simulink library "halin"  (R2021b)
settings: Solver=VariableStepAuto  StartTime=0.0  StopTime=10.0  RelTol=1e-3
undefined symbols (not defined in the file): TRUE
libraries: FVT_lib x177, hcu_lib x55
(part 14 of 17)

== system halin/HAL_IN/CAN2/IVI3/IVICLBlowerYSta ==
  IVI_CLBlower_Y_Sta : Inport
  UnitConverter : DataTypeConversion  OutDataTypeStr=uint8
  VHAL_IVICLBlowerYSta_pct : Outport
  wires:
  UnitConverter/1 -> VHAL_IVICLBlowerYSta_pct/1
  IVI_CLBlower_Y_Sta/1 -> UnitConverter/1

== system halin/HAL_IN/CAN2/IVI3/IVICLBlowerZSta ==
  IVI_CLBlower_Z_Sta : Inport
  UnitConverter : DataTypeConversion  OutDataTypeStr=uint8
  VHAL_IVICLBlowerZSta_pct : Outport
  wires:
  UnitConverter/1 -> VHAL_IVICLBlowerZSta_pct/1
  IVI_CLBlower_Z_Sta/1 -> UnitConverter/1

== system halin/HAL_IN/CAN2/IVI3/IVICRBlowerYSta ==
  IVI_CRBlower_Y_Sta : Inport
  UnitConverter : DataTypeConversion  OutDataTypeStr=uint8
  VHAL_IVICRBlowerYSta_pct : Outport
  wires:
  UnitConverter/1 -> VHAL_IVICRBlowerYSta_pct/1
  IVI_CRBlower_Y_Sta/1 -> UnitConverter/1

== system halin/HAL_IN/CAN2/IVI3/IVICRBlowerZSta ==
  IVI_CRBlower_Z_Sta : Inport
  UnitConverter : DataTypeConversion  OutDataTypeStr=uint8
  VHAL_IVICRBlowerZSta_pct : Outport
  wires:
  UnitConverter/1 -> VHAL_IVICRBlowerZSta_pct/1
  IVI_CRBlower_Z_Sta/1 -> UnitConverter/1

== system halin/HAL_IN/CAN2/IVI3/IVIDrBlowerModeSta ==
  IVI_DrBlower_Mode_Sta : Inport
  UnitConverter : DataTypeConversion  OutDataTypeStr=uint8
  VHAL_IVIDrBlowerModeSta_enum : Outport
  wires:
  UnitConverter/1 -> VHAL_IVIDrBlowerModeSta_enum/1
  IVI_DrBlower_Mode_Sta/1 -> UnitConverter/1

== system halin/HAL_IN/CAN2/IVI3/IVIDrBlowerYSta ==
  IVI_DrBlower_Y_Sta : Inport
  UnitConverter : DataTypeConversion  OutDataTypeStr=uint8
  VHAL_IVIDrBlowerYSta_pct : Outport
  wires:
  UnitConverter/1 -> VHAL_IVIDrBlowerYSta_pct/1
  IVI_DrBlower_Y_Sta/1 -> UnitConverter/1

== system halin/HAL_IN/CAN2/IVI3/IVIDrBlowerZSta ==
  IVI_DrBlower_Z_Sta : Inport
  UnitConverter : DataTypeConversion  OutDataTypeStr=uint8
  VHAL_IVIDrBlowerZSta_pct : Outport
  wires:
  UnitConverter/1 -> VHAL_IVIDrBlowerZSta_pct/1
  IVI_DrBlower_Z_Sta/1 -> UnitConverter/1

== system halin/HAL_IN/CAN2/IVI3/IVILSEATventCmd ==
  IVI_LSEATvent_Cmd : Inport
  UnitConverter : DataTypeConversion  OutDataTypeStr=uint8
  VHAL_IVILSEATventCmd_enum : Outport
  wires:
  UnitConverter/1 -> VHAL_IVILSEATventCmd_enum/1
  IVI_LSEATvent_Cmd/1 -> UnitConverter/1

== system halin/HAL_IN/CAN2/IVI3/IVIMLFMostCmd ==
  IVI_MLFMost_Cmd : Inport
  UnitConverter : DataTypeConversion  OutDataTypeStr=uint8
  VHAL_IVIMLFMostCmd_flg : Outport
  wires:
  UnitConverter/1 -> VHAL_IVIMLFMostCmd_flg/1
  IVI_MLFMost_Cmd/1 -> UnitConverter/1

== system halin/HAL_IN/CAN2/IVI3/IVIMLFootLiftCmd ==
  IVI_MLFootLift_Cmd : Inport
  UnitConverter : DataTypeConversion  OutDataTypeStr=uint8
  VHAL_IVIMLFootLiftCmd_enum : Outport
  wires:
  UnitConverter/1 -> VHAL_IVIMLFootLiftCmd_enum/1
  IVI_MLFootLift_Cmd/1 -> UnitConverter/1

== system halin/HAL_IN/CAN2/IVI3/IVIMLNapModeCmd ==
  IVI_MLNapMode_Cmd : Inport
  UnitConverter : DataTypeConversion  OutDataTypeStr=uint8
  VHAL_IVIMLNapModeCmd_flg : Outport
  wires:
  UnitConverter/1 -> VHAL_IVIMLNapModeCmd_flg/1
  IVI_MLNapMode_Cmd/1 -> UnitConverter/1

== system halin/HAL_IN/CAN2/IVI3/IVIMLReclinerCmd ==
  IVI_MLRecliner_Cmd : Inport
  UnitConverter : DataTypeConversion  OutDataTypeStr=uint8
  VHAL_IVIMLReclinerCmd_enum : Outport
  wires:
  UnitConverter/1 -> VHAL_IVIMLReclinerCmd_enum/1
  IVI_MLRecliner_Cmd/1 -> UnitConverter/1

== system halin/HAL_IN/CAN2/IVI3/IVIMLRestoreCmd ==
  IVI_MLRestore_Cmd : Inport
  UnitConverter : DataTypeConversion  OutDataTypeStr=uint8
  VHAL_IVIMLRestoreCmd_flg : Outport
  wires:
  UnitConverter/1 -> VHAL_IVIMLRestoreCmd_flg/1
  IVI_MLRestore_Cmd/1 -> UnitConverter/1

== system halin/HAL_IN/CAN2/IVI3/IVIMLSEATventCmd ==
  IVI_MLSEATvent_Cmd : Inport
  UnitConverter : DataTypeConversion  OutDataTypeStr=uint8
  VHAL_IVIMLSEATventCmd_enum : Outport
  wires:
  UnitConverter/1 -> VHAL_IVIMLSEATventCmd_enum/1
  IVI_MLSEATvent_Cmd/1 -> UnitConverter/1

== system halin/HAL_IN/CAN2/IVI3/IVIMLSeatLiftCmd ==
  IVI_MLSeatLift_Cmd : Inport
  UnitConverter : DataTypeConversion  OutDataTypeStr=uint8
  VHAL_IVIMLSeatLiftCmd_enum : Outport
  wires:
  UnitConverter/1 -> VHAL_IVIMLSeatLiftCmd_enum/1
  IVI_MLSeatLift_Cmd/1 -> UnitConverter/1

== system halin/HAL_IN/CAN2/IVI3/IVIMLSldRestoreCmd ==
  IVI_MLSldRestore_Cmd : Inport
  UnitConverter : DataTypeConversion  OutDataTypeStr=uint8
  VHAL_IVIMLSldRestoreCmd_flg : Outport
  wires:
  UnitConverter/1 -> VHAL_IVIMLSldRestoreCmd_flg/1
  IVI_MLSldRestore_Cmd/1 -> UnitConverter/1

== system halin/HAL_IN/CAN2/IVI3/IVIMLSliderCmd ==
  IVI_MLSlider_Cmd : Inport
  UnitConverter : DataTypeConversion  OutDataTypeStr=uint8
  VHAL_IVIMLSliderCmd_enum : Outport
  wires:
  UnitConverter/1 -> VHAL_IVIMLSliderCmd_enum/1
  IVI_MLSlider_Cmd/1 -> UnitConverter/1

== system halin/HAL_IN/CAN2/IVI3/IVIMLZeroGravityCmd ==
  IVI_MLZeroGravity_Cmd : Inport
  UnitConverter : DataTypeConversion  OutDataTypeStr=uint8
  VHAL_IVIMLZeroGravityCmd_flg : Outport
  wires:
  UnitConverter/1 -> VHAL_IVIMLZeroGravityCmd_flg/1
  IVI_MLZeroGravity_Cmd/1 -> UnitConverter/1

== system halin/HAL_IN/CAN2/IVI3/IVIMRFMostCmd ==
  IVI_MRFMost_Cmd : Inport
  UnitConverter : DataTypeConversion  OutDataTypeStr=uint8
  VHAL_IVIMRFMostCmd_flg : Outport
  wires:
  UnitConverter/1 -> VHAL_IVIMRFMostCmd_flg/1
  IVI_MRFMost_Cmd/1 -> UnitConverter/1

== system halin/HAL_IN/CAN2/IVI3/IVIMRFootLiftCmd ==
  IVI_MRFootLift_Cmd : Inport
  UnitConverter : DataTypeConversion  OutDataTypeStr=uint8
  VHAL_IVIMRFootLiftCmd_enum : Outport
  wires:
  UnitConverter/1 -> VHAL_IVIMRFootLiftCmd_enum/1
  IVI_MRFootLift_Cmd/1 -> UnitConverter/1

== system halin/HAL_IN/CAN2/IVI3/IVIMRNapModeCmd ==
  IVI_MRNapMode_Cmd : Inport
  UnitConverter : DataTypeConversion  OutDataTypeStr=uint8
  VHAL_IVIMRNapModeCmd_flg : Outport
  wires:
  UnitConverter/1 -> VHAL_IVIMRNapModeCmd_flg/1
  IVI_MRNapMode_Cmd/1 -> UnitConverter/1

== system halin/HAL_IN/CAN2/IVI3/IVIMRReclinerCmd ==
  IVI_MRRecliner_Cmd : Inport
  UnitConverter : DataTypeConversion  OutDataTypeStr=uint8
  VHAL_IVIMRReclinerCmd_enum : Outport
  wires:
  UnitConverter/1 -> VHAL_IVIMRReclinerCmd_enum/1
  IVI_MRRecliner_Cmd/1 -> UnitConverter/1

== system halin/HAL_IN/CAN2/IVI3/IVIMRRestoreCmd ==
  IVI_MRRestore_Cmd : Inport
  UnitConverter : DataTypeConversion  OutDataTypeStr=uint8
  VHAL_IVIMRRestoreCmd_flg : Outport
  wires:
  UnitConverter/1 -> VHAL_IVIMRRestoreCmd_flg/1
  IVI_MRRestore_Cmd/1 -> UnitConverter/1

== system halin/HAL_IN/CAN2/IVI3/IVIMRSEATventCmd ==
  IVI_MRSEATvent_Cmd : Inport
  UnitConverter : DataTypeConversion  OutDataTypeStr=uint8
  VHAL_IVIMRSEATventCmd_enum : Outport
  wires:
  UnitConverter/1 -> VHAL_IVIMRSEATventCmd_enum/1
  IVI_MRSEATvent_Cmd/1 -> UnitConverter/1

== system halin/HAL_IN/CAN2/IVI3/IVIMRSeatLiftCmd ==
  IVI_MRSeatLift_Cmd : Inport
  UnitConverter : DataTypeConversion  OutDataTypeStr=uint8
  VHAL_IVIMRSeatLiftCmd_enum : Outport
  wires:
  UnitConverter/1 -> VHAL_IVIMRSeatLiftCmd_enum/1
  IVI_MRSeatLift_Cmd/1 -> UnitConverter/1

== system halin/HAL_IN/CAN2/IVI3/IVIMRSldRestoreCmd ==
  IVI_MRSldRestore_Cmd : Inport
  UnitConverter : DataTypeConversion  OutDataTypeStr=uint8
  VHAL_IVIMRSldRestoreCmd_flg : Outport
  wires:
  UnitConverter/1 -> VHAL_IVIMRSldRestoreCmd_flg/1
  IVI_MRSldRestore_Cmd/1 -> UnitConverter/1

== system halin/HAL_IN/CAN2/IVI3/IVIMRSliderCmd ==
  IVI_MRSlider_Cmd : Inport
  UnitConverter : DataTypeConversion  OutDataTypeStr=uint8
  VHAL_IVIMRSliderCmd_enum : Outport
  wires:
  UnitConverter/1 -> VHAL_IVIMRSliderCmd_enum/1
  IVI_MRSlider_Cmd/1 -> UnitConverter/1

== system halin/HAL_IN/CAN2/IVI3/IVIMRZeroGravityCmd ==
  IVI_MRZeroGravity_Cmd : Inport
  UnitConverter : DataTypeConversion  OutDataTypeStr=uint8
  VHAL_IVIMRZeroGravityCmd_flg : Outport
  wires:
  UnitConverter/1 -> VHAL_IVIMRZeroGravityCmd_flg/1
  IVI_MRZeroGravity_Cmd/1 -> UnitConverter/1

== system halin/HAL_IN/CAN2/IVI3/IVIPsBlowerModeSta ==
  IVI_PsBlower_Mode_Sta : Inport
  UnitConverter : DataTypeConversion  OutDataTypeStr=uint8
  VHAL_IVIPsBlowerModeSta_enum : Outport
  wires:
  UnitConverter/1 -> VHAL_IVIPsBlowerModeSta_enum/1
  IVI_PsBlower_Mode_Sta/1 -> UnitConverter/1

== system halin/HAL_IN/CAN2/IVI3/IVIPsBlowerYSta ==
  IVI_PsBlower_Y_Sta : Inport
  UnitConverter : DataTypeConversion  OutDataTypeStr=uint8
  VHAL_IVIPsBlowerYSta_pct : Outport
  wires:
  UnitConverter/1 -> VHAL_IVIPsBlowerYSta_pct/1
  IVI_PsBlower_Y_Sta/1 -> UnitConverter/1

== system halin/HAL_IN/CAN2/IVI3/IVIPsBlowerZSta ==
  IVI_PsBlower_Z_Sta : Inport
  UnitConverter : DataTypeConversion  OutDataTypeStr=uint8
  VHAL_IVIPsBlowerZSta_pct : Outport
  wires:
  UnitConverter/1 -> VHAL_IVIPsBlowerZSta_pct/1
  IVI_PsBlower_Z_Sta/1 -> UnitConverter/1

== system halin/HAL_IN/CAN2/IVI3/IVIRSEATventCmd ==
  IVI_RSEATvent_Cmd : Inport
  UnitConverter : DataTypeConversion  OutDataTypeStr=uint8
  VHAL_IVIRSEATventCmd_enum : Outport
  wires:
  UnitConverter/1 -> VHAL_IVIRSEATventCmd_enum/1
  IVI_RSEATvent_Cmd/1 -> UnitConverter/1

== system halin/HAL_IN/CAN2/METER1/METERKPHCalcu ==
  METER_KPH_Calcu : Inport
  UnitConverter : DataTypeConversion  OutDataTypeStr=uint8
  VHAL_METERKPHCalcu_kph : Outport
  wires:
  UnitConverter/1 -> VHAL_METERKPHCalcu_kph/1
  METER_KPH_Calcu/1 -> UnitConverter/1

== system halin/HAL_IN/CAN2/METER1/ODOMETER ==
  ODOMETER : Inport
  UnitConverter : DataTypeConversion  OutDataTypeStr=uint32
  convert_in : FVT_lib/hal/convert_in  gain=0.1  offset=0
  VHAL_ODOMETER_km : Outport
  wires:
  convert_in/1 -> VHAL_ODOMETER_km/1
  UnitConverter/1 -> convert_in/1
  ODOMETER/1 -> UnitConverter/1

== system halin/HAL_IN/CAN3/BMS1/BMSChckSum1 ==
  BMSChckSum_1 : Inport
  UnitConverter : DataTypeConversion  OutDataTypeStr=uint8
  VHAL_BMSChckSum1_enum : Outport
  wires:
  UnitConverter/1 -> VHAL_BMSChckSum1_enum/1
  BMSChckSum_1/1 -> UnitConverter/1

== system halin/HAL_IN/CAN3/BMS1/BMSRolCnct1 ==
  BMSRolCnct_1 : Inport
  UnitConverter : DataTypeConversion  OutDataTypeStr=uint8
  VHAL_BMSRolCnct1_enum : Outport
  wires:
  UnitConverter/1 -> VHAL_BMSRolCnct1_enum/1
  BMSRolCnct_1/1 -> UnitConverter/1

== system halin/HAL_IN/CAN3/BMS1/HVBPwrAvailChrg ==
  HVBPwrAvailChrg : Inport
  UnitConverter : DataTypeConversion  OutDataTypeStr=uint16
  convert_in : FVT_lib/hal/convert_in  gain=0.2  offset=0
  VHAL_HVBPwrAvailChrg_kW : Outport
  wires:
  convert_in/1 -> VHAL_HVBPwrAvailChrg_kW/1
  UnitConverter/1 -> convert_in/1
  HVBPwrAvailChrg/1 -> UnitConverter/1

== system halin/HAL_IN/CAN3/BMS1/HVBPwrAvailChrg30 ==
  HVBPwrAvailChrg30 : Inport
  UnitConverter : DataTypeConversion  OutDataTypeStr=uint16
  convert_in : FVT_lib/hal/convert_in  gain=0.2  offset=0
  VHAL_HVBPwrAvailChrg30_kW : Outport
  wires:
  convert_in/1 -> VHAL_HVBPwrAvailChrg30_kW/1
  UnitConverter/1 -> convert_in/1
  HVBPwrAvailChrg30/1 -> UnitConverter/1

== system halin/HAL_IN/CAN3/BMS1/HVBPwrAvailChrg60 ==
  HVBPwrAvailChrg60 : Inport
  UnitConverter : DataTypeConversion  OutDataTypeStr=uint16
  convert_in : FVT_lib/hal/convert_in  gain=0.2  offset=0
  VHAL_HVBPwrAvailChrg60_kW : Outport
  wires:
  convert_in/1 -> VHAL_HVBPwrAvailChrg60_kW/1
  UnitConverter/1 -> convert_in/1
  HVBPwrAvailChrg60/1 -> UnitConverter/1

== system halin/HAL_IN/CAN3/BMS1/HVBPwrAvailDchrg ==
  HVBPwrAvailDchrg : Inport
  UnitConverter : DataTypeConversion  OutDataTypeStr=uint16
  convert_in : FVT_lib/hal/convert_in  gain=0.2  offset=0
  VHAL_HVBPwrAvailDchrg_kW : Outport
  wires:
  convert_in/1 -> VHAL_HVBPwrAvailDchrg_kW/1
  UnitConverter/1 -> convert_in/1
  HVBPwrAvailDchrg/1 -> UnitConverter/1

== system halin/HAL_IN/CAN3/BMS1/HVBPwrAvailDchrg30 ==
  HVBPwrAvailDchrg30 : Inport
  UnitConverter : DataTypeConversion  OutDataTypeStr=uint16
  convert_in : FVT_lib/hal/convert_in  gain=0.2  offset=0
  VHAL_HVBPwrAvailDchrg30_kW : Outport
  wires:
  convert_in/1 -> VHAL_HVBPwrAvailDchrg30_kW/1
  UnitConverter/1 -> convert_in/1
  HVBPwrAvailDchrg30/1 -> UnitConverter/1

== system halin/HAL_IN/CAN3/BMS1/HVBPwrAvailDchrg60 ==
  HVBPwrAvailDchrg60 : Inport
  UnitConverter : DataTypeConversion  OutDataTypeStr=uint16
  convert_in : FVT_lib/hal/convert_in  gain=0.2  offset=0
  VHAL_HVBPwrAvailDchrg60_kW : Outport
  wires:
  convert_in/1 -> VHAL_HVBPwrAvailDchrg60_kW/1
  UnitConverter/1 -> convert_in/1
  HVBPwrAvailDchrg60/1 -> UnitConverter/1

== system halin/HAL_IN/CAN3/BMS1/HVBattCurr ==
  HVBattCurr : Inport
  UnitConverter : DataTypeConversion  OutDataTypeStr=uint16
  convert_in : FVT_lib/hal/convert_in  gain=0.1  offset=-1000
  VHAL_HVBattCurr_A : Outport
  wires:
  convert_in/1 -> VHAL_HVBattCurr_A/1
  UnitConverter/1 -> convert_in/1
  HVBattCurr/1 -> UnitConverter/1

== system halin/HAL_IN/CAN3/BMS1/HVBattVolt ==
  HVBattVolt : Inport
  UnitConverter : DataTypeConversion  OutDataTypeStr=uint16
  convert_in : FVT_lib/hal/convert_in  gain=0.1  offset=0
  VHAL_HVBattVolt_V : Outport
  wires:
  convert_in/1 -> VHAL_HVBattVolt_V/1
  UnitConverter/1 -> convert_in/1
  HVBattVolt/1 -> UnitConverter/1

== system halin/HAL_IN/CAN3/BMS3/ACChrgCurrDis ==
  ACChrgCurrDis : Inport
  UnitConverter : DataTypeConversion  OutDataTypeStr=uint16
  convert_in : FVT_lib/hal/convert_in  gain=0.1  offset=-1000
  VHAL_ACChrgCurrDis_A : Outport
  wires:
  convert_in/1 -> VHAL_ACChrgCurrDis_A/1
  UnitConverter/1 -> convert_in/1
  ACChrgCurrDis/1 -> UnitConverter/1

== system halin/HAL_IN/CAN3/BMS3/FireDetErr ==
  FireDetErr : Inport
  UnitConverter : DataTypeConversion  OutDataTypeStr=uint8
  VHAL_FireDetErr_flg : Outport
  wires:
  UnitConverter/1 -> VHAL_FireDetErr_flg/1
  FireDetErr/1 -> UnitConverter/1

== system halin/HAL_IN/CAN3/BMS3/HVBChrgPwr ==
  HVBChrgPwr : Inport
  UnitConverter : DataTypeConversion  OutDataTypeStr=uint16
  convert_in : FVT_lib/hal/convert_in  gain=0.1  offset=0
  VHAL_HVBChrgPwr_kWh : Outport
  wires:
  convert_in/1 -> VHAL_HVBChrgPwr_kWh/1
  UnitConverter/1 -> convert_in/1
  HVBChrgPwr/1 -> UnitConverter/1

== system halin/HAL_IN/CAN3/BMS3/HVBChrgPwrTotal ==
  HVBChrgPwrTotal : Inport
  UnitConverter : DataTypeConversion  OutDataTypeStr=uint32
  VHAL_HVBChrgPwrTotal_kWh : Outport
  wires:
  UnitConverter/1 -> VHAL_HVBChrgPwrTotal_kWh/1
  HVBChrgPwrTotal/1 -> UnitConverter/1

== system halin/HAL_IN/CAN3/BMS3/HVBDrvPwr ==
  HVBDrvPwr : Inport
  UnitConverter : DataTypeConversion  OutDataTypeStr=uint16
  convert_in : FVT_lib/hal/convert_in  gain=0.1  offset=0
  VHAL_HVBDrvPwr_kWh : Outport
  wires:
  convert_in/1 -> VHAL_HVBDrvPwr_kWh/1
  UnitConverter/1 -> convert_in/1
  HVBDrvPwr/1 -> UnitConverter/1

== system halin/HAL_IN/CAN3/BMS3/HVBDrvPwrTotal ==
  HVBDrvPwrTotal : Inport
  UnitConverter : DataTypeConversion  OutDataTypeStr=uint32
  VHAL_HVBDrvPwrTotal_kWh : Outport
  wires:
  UnitConverter/1 -> VHAL_HVBDrvPwrTotal_kWh/1
  HVBDrvPwrTotal/1 -> UnitConverter/1

== system halin/HAL_IN/CAN3/BMS3/HVBFullChrgPwr ==
  HVBFullChrgPwr : Inport
  UnitConverter : DataTypeConversion  OutDataTypeStr=uint16
  convert_in : FVT_lib/hal/convert_in  gain=0.1  offset=0
  VHAL_HVBFullChrgPwr_kWh : Outport
  wires:
  convert_in/1 -> VHAL_HVBFullChrgPwr_kWh/1
  UnitConverter/1 -> convert_in/1
  HVBFullChrgPwr/1 -> UnitConverter/1

== system halin/HAL_IN/CAN3/BMS3/HVBIsoImpedenceN ==
  HVBIsoImpedenceN : Inport
  UnitConverter : DataTypeConversion  OutDataTypeStr=uint16
  convert_in : FVT_lib/hal/convert_in  gain=0.01  offset=0
  VHAL_HVBIsoImpedenceN_Megaohm : Outport
  wires:
  convert_in/1 -> VHAL_HVBIsoImpedenceN_Megaohm/1
  UnitConverter/1 -> convert_in/1
  HVBIsoImpedenceN/1 -> UnitConverter/1

== system halin/HAL_IN/CAN3/BMS3/HVBIsoImpedenceP ==
  HVBIsoImpedenceP : Inport
  UnitConverter : DataTypeConversion  OutDataTypeStr=uint16
  convert_in : FVT_lib/hal/convert_in  gain=0.01  offset=0
  VHAL_HVBIsoImpedenceP_Megaohm : Outport
  wires:
  convert_in/1 -> VHAL_HVBIsoImpedenceP_Megaohm/1
  UnitConverter/1 -> convert_in/1
  HVBIsoImpedenceP/1 -> UnitConverter/1

== system halin/HAL_IN/CAN3/BMS3/HVBSOH ==
  HVBSOH : Inport
  UnitConverter : DataTypeConversion  OutDataTypeStr=uint8
  convert_in : FVT_lib/hal/convert_in  gain=0.4  offset=0
  VHAL_HVBSOH_pct : Outport
  wires:
  convert_in/1 -> VHAL_HVBSOH_pct/1
  UnitConverter/1 -> convert_in/1
  HVBSOH/1 -> UnitConverter/1

== system halin/HAL_IN/CAN3/BMS3/HVBattErr ==
  HVBattErr : Inport
  UnitConverter : DataTypeConversion  OutDataTypeStr=uint8
  VHAL_HVBattErr_flg : Outport
  wires:
  UnitConverter/1 -> VHAL_HVBattErr_flg/1
  HVBattErr/1 -> UnitConverter/1

== system halin/HAL_IN/CAN3/BMS3/HVBattPackVolt ==
  HVBattPackVolt : Inport
  UnitConverter : DataTypeConversion  OutDataTypeStr=uint16
  convert_in : FVT_lib/hal/convert_in  gain=0.1  offset=0
  VHAL_HVBattPackVolt_V : Outport
  wires:
  convert_in/1 -> VHAL_HVBattPackVolt_V/1
  UnitConverter/1 -> convert_in/1
  HVBattPackVolt/1 -> UnitConverter/1

== system halin/HAL_IN/CAN3/BMS3/HVBattSOC ==
  HVBattSOC : Inport
  UnitConverter : DataTypeConversion  OutDataTypeStr=uint8
  convert_in : FVT_lib/hal/convert_in  gain=0.4  offset=0
  VHAL_HVBattSOC_pct : Outport
  wires:
  convert_in/1 -> VHAL_HVBattSOC_pct/1
  UnitConverter/1 -> convert_in/1
  HVBattSOC/1 -> UnitConverter/1

== system halin/HAL_IN/CAN3/BMS3/HVBattSOCDis ==
  HVBattSOCDis : Inport
  UnitConverter : DataTypeConversion  OutDataTypeStr=uint8
  convert_in : FVT_lib/hal/convert_in  gain=0.4  offset=0
  VHAL_HVBattSOCDis_pct : Outport
  wires:
  convert_in/1 -> VHAL_HVBattSOCDis_pct/1
  UnitConverter/1 -> convert_in/1
  HVBattSOCDis/1 -> UnitConverter/1

== system halin/HAL_IN/CAN3/BMS3/RemainChrgTime ==
  RemainChrgTime : Inport
  UnitConverter : DataTypeConversion  OutDataTypeStr=uint16
  VHAL_RemainChrgTime_min : Outport
  wires:
  UnitConverter/1 -> VHAL_RemainChrgTime_min/1
  RemainChrgTime/1 -> UnitConverter/1

== system halin/HAL_IN/CAN3/BMS4/CellTempAvg ==
  CellTempAvg : Inport
  UnitConverter : DataTypeConversion  OutDataTypeStr=uint8
  convert_in : FVT_lib/hal/convert_in  gain=1  offset=-40
  VHAL_CellTempAvg_C : Outport
  wires:
  convert_in/1 -> VHAL_CellTempAvg_C/1
  UnitConverter/1 -> convert_in/1
  CellTempAvg/1 -> UnitConverter/1

== system halin/HAL_IN/CAN3/BMS4/HVBCellVoltMax ==
  HVBCellVoltMax : Inport
  UnitConverter : DataTypeConversion  OutDataTypeStr=uint16
  VHAL_HVBCellVoltMax_mV : Outport
  wires:
  UnitConverter/1 -> VHAL_HVBCellVoltMax_mV/1
  HVBCellVoltMax/1 -> UnitConverter/1

== system halin/HAL_IN/CAN3/BMS4/HVBCellVoltMin ==
  HVBCellVoltMin : Inport
  UnitConverter : DataTypeConversion  OutDataTypeStr=uint16
  VHAL_HVBCellVoltMin_mV : Outport
  wires:
  UnitConverter/1 -> VHAL_HVBCellVoltMin_mV/1
  HVBCellVoltMin/1 -> UnitConverter/1

== system halin/HAL_IN/CAN3/BMS4/HVBMTempMax ==
  HVBMTempMax : Inport
  UnitConverter : DataTypeConversion  OutDataTypeStr=uint8
  convert_in : FVT_lib/hal/convert_in  gain=1  offset=-40
  VHAL_HVBMTempMax_C : Outport
  wires:
  convert_in/1 -> VHAL_HVBMTempMax_C/1
  UnitConverter/1 -> convert_in/1
  HVBMTempMax/1 -> UnitConverter/1

== system halin/HAL_IN/CAN3/BMS4/HVBMTempMin ==
  HVBMTempMin : Inport
  UnitConverter : DataTypeConversion  OutDataTypeStr=uint8
  convert_in : FVT_lib/hal/convert_in  gain=1  offset=-40
  VHAL_HVBMTempMin_C : Outport
  wires:
  convert_in/1 -> VHAL_HVBMTempMin_C/1
  UnitConverter/1 -> convert_in/1
  HVBMTempMin/1 -> UnitConverter/1

== system halin/HAL_IN/CAN3/BMS4/MaxCellTempNum ==
  MaxCellTemp_Num : Inport
  UnitConverter : DataTypeConversion  OutDataTypeStr=uint8
  VHAL_MaxCellTempNum_enum : Outport
  wires:
  UnitConverter/1 -> VHAL_MaxCellTempNum_enum/1
  MaxCellTemp_Num/1 -> UnitConverter/1

== system halin/HAL_IN/CAN3/BMS4/MaxCellVoltNum ==
  MaxCellVolt_Num : Inport
  UnitConverter : DataTypeConversion  OutDataTypeStr=uint8
  VHAL_MaxCellVoltNum_enum : Outport
  wires:
  UnitConverter/1 -> VHAL_MaxCellVoltNum_enum/1
  MaxCellVolt_Num/1 -> UnitConverter/1

== system halin/HAL_IN/CAN3/BMS4/MinCellTempNum ==
  MinCellTemp_Num : Inport
  UnitConverter : DataTypeConversion  OutDataTypeStr=uint8
  VHAL_MinCellTempNum_enum : Outport
  wires:
  UnitConverter/1 -> VHAL_MinCellTempNum_enum/1
  MinCellTemp_Num/1 -> UnitConverter/1

== system halin/HAL_IN/CAN3/BMS4/MinCellVoltNum ==
  MinCellVolt_Num : Inport
  UnitConverter : DataTypeConversion  OutDataTypeStr=uint8
  VHAL_MinCellVoltNum_enum : Outport
  wires:
  UnitConverter/1 -> VHAL_MinCellVoltNum_enum/1
  MinCellVolt_Num/1 -> UnitConverter/1

== system halin/HAL_IN/CAN3/BMS5/HVInVolt ==
  HVInVolt : Inport
  UnitConverter : DataTypeConversion  OutDataTypeStr=uint16
  convert_in : FVT_lib/hal/convert_in  gain=0.1  offset=0
  VHAL_HVInVolt_V : Outport
  wires:
  convert_in/1 -> VHAL_HVInVolt_V/1
  UnitConverter/1 -> convert_in/1
  HVInVolt/1 -> UnitConverter/1

== system halin/HAL_IN/CAN3/BMS5/LVBattDet12V ==
  LVBattDet12V : Inport
  UnitConverter : DataTypeConversion  OutDataTypeStr=uint8
  convert_in : FVT_lib/hal/convert_in  gain=0.1  offset=0
  VHAL_LVBattDet12V_V : Outport
  wires:
  convert_in/1 -> VHAL_LVBattDet12V_V/1
  UnitConverter/1 -> convert_in/1
  LVBattDet12V/1 -> UnitConverter/1

== system halin/HAL_IN/CAN3/BMS5/OBCACCSLimit ==
  OBCACCSLimit : Inport
  UnitConverter : DataTypeConversion  OutDataTypeStr=uint8
  VHAL_OBCACCSLimit_A : Outport
  wires:
  UnitConverter/1 -> VHAL_OBCACCSLimit_A/1
  OBCACCSLimit/1 -> UnitConverter/1

== system halin/HAL_IN/CAN3/BMS5/OBCDCCurLm ==
  OBCDCCurLm : Inport
  UnitConverter : DataTypeConversion  OutDataTypeStr=uint16
  convert_in : FVT_lib/hal/convert_in  gain=0.1  offset=-25.5
  VHAL_OBCDCCurLm_A : Outport
  wires:
  convert_in/1 -> VHAL_OBCDCCurLm_A/1
  UnitConverter/1 -> convert_in/1
  OBCDCCurLm/1 -> UnitConverter/1

== system halin/HAL_IN/CAN3/BMS5/OBCDCVoltLm ==
  OBCDCVoltLm : Inport
  UnitConverter : DataTypeConversion  OutDataTypeStr=uint16
  convert_in : FVT_lib/hal/convert_in  gain=0.1  offset=0
  VHAL_OBCDCVoltLm_V : Outport
  wires:
  convert_in/1 -> VHAL_OBCDCVoltLm_V/1
  UnitConverter/1 -> convert_in/1
  OBCDCVoltLm/1 -> UnitConverter/1

== system halin/HAL_IN/CAN3/BMS6/BMSChckSum ==
  BMSChckSum : Inport
  UnitConverter : DataTypeConversion  OutDataTypeStr=uint8
  VHAL_BMSChckSum_enum : Outport
  wires:
  UnitConverter/1 -> VHAL_BMSChckSum_enum/1
  BMSChckSum/1 -> UnitConverter/1

== system halin/HAL_IN/CAN3/BMS6/BMSREADY ==
  BMS_READY : Inport
  UnitConverter : DataTypeConversion  OutDataTypeStr=uint8
  VHAL_BMSREADY_flg : Outport
  wires:
  UnitConverter/1 -> VHAL_BMSREADY_flg/1
  BMS_READY/1 -> UnitConverter/1

== system halin/HAL_IN/CAN3/BMS6/BMSRolCnct ==
  BMSRolCnct : Inport
  UnitConverter : DataTypeConversion  OutDataTypeStr=uint8
  VHAL_BMSRolCnct_enum : Outport
  wires:
  UnitConverter/1 -> VHAL_BMSRolCnct_enum/1
  BMSRolCnct/1 -> UnitConverter/1

== system halin/HAL_IN/CAN3/BMS6/BMSWarn1 ==
  BMS_Warn_1 : Inport
  UnitConverter : DataTypeConversion  OutDataTypeStr=uint8
  VHAL_BMSWarn1_flg : Outport
  wires:
  UnitConverter/1 -> VHAL_BMSWarn1_flg/1
  BMS_Warn_1/1 -> UnitConverter/1

== system halin/HAL_IN/CAN3/BMS6/BMSWarn2 ==
  BMS_Warn_2 : Inport
  UnitConverter : DataTypeConversion  OutDataTypeStr=uint8
  VHAL_BMSWarn2_flg : Outport
  wires:
  UnitConverter/1 -> VHAL_BMSWarn2_flg/1
  BMS_Warn_2/1 -> UnitConverter/1

== system halin/HAL_IN/CAN3/BMS6/BMSWarn3 ==
  BMS_Warn_3 : Inport
  UnitConverter : DataTypeConversion  OutDataTypeStr=uint8
  VHAL_BMSWarn3_flg : Outport
  wires:
  UnitConverter/1 -> VHAL_BMSWarn3_flg/1
  BMS_Warn_3/1 -> UnitConverter/1

== system halin/HAL_IN/CAN3/BMS6/BMSWarn4 ==
  BMS_Warn_4 : Inport
  UnitConverter : DataTypeConversion  OutDataTypeStr=uint8
  VHAL_BMSWarn4_flg : Outport
  wires:
  UnitConverter/1 -> VHAL_BMSWarn4_flg/1
  BMS_Warn_4/1 -> UnitConverter/1

== system halin/HAL_IN/CAN3/BMS6/BMSWarn5 ==
  BMS_Warn_5 : Inport
  UnitConverter : DataTypeConversion  OutDataTypeStr=uint8
  VHAL_BMSWarn5_flg : Outport
  wires:
  UnitConverter/1 -> VHAL_BMSWarn5_flg/1
  BMS_Warn_5/1 -> UnitConverter/1

== system halin/HAL_IN/CAN3/BMS6/BMSWarn6 ==
  BMS_Warn_6 : Inport
  UnitConverter : DataTypeConversion  OutDataTypeStr=uint8
  VHAL_BMSWarn6_flg : Outport
  wires:
  UnitConverter/1 -> VHAL_BMSWarn6_flg/1
  BMS_Warn_6/1 -> UnitConverter/1

== system halin/HAL_IN/CAN3/BMS6/BMSWarn7 ==
  BMS_Warn_7 : Inport
  UnitConverter : DataTypeConversion  OutDataTypeStr=uint8
  VHAL_BMSWarn7_flg : Outport
  wires:
  UnitConverter/1 -> VHAL_BMSWarn7_flg/1
  BMS_Warn_7/1 -> UnitConverter/1

== system halin/HAL_IN/CAN3/BMS6/BMSWarn8 ==
  BMS_Warn_8 : Inport
  UnitConverter : DataTypeConversion  OutDataTypeStr=uint8
  VHAL_BMSWarn8_flg : Outport
  wires:
  UnitConverter/1 -> VHAL_BMSWarn8_flg/1
  BMS_Warn_8/1 -> UnitConverter/1

== system halin/HAL_IN/CAN3/BMS6/ChrgInLockReq ==
  ChrgInLockReq : Inport
  UnitConverter : DataTypeConversion  OutDataTypeStr=uint8
  VHAL_ChrgInLockReq_enum : Outport
  wires:
  UnitConverter/1 -> VHAL_ChrgInLockReq_enum/1
  ChrgInLockReq/1 -> UnitConverter/1

== system halin/HAL_IN/CAN3/BMS6/ChrgPlugSta ==
  ChrgPlugSta : Inport
  UnitConverter : DataTypeConversion  OutDataTypeStr=uint8
  VHAL_ChrgPlugSta_enum : Outport
  wires:
  UnitConverter/1 -> VHAL_ChrgPlugSta_enum/1
  ChrgPlugSta/1 -> UnitConverter/1

== system halin/HAL_IN/CAN3/BMS6/DisChrgPlugErr ==
  DisChrgPlugErr : Inport
  UnitConverter : DataTypeConversion  OutDataTypeStr=uint8
  VHAL_DisChrgPlugErr_enum : Outport
  wires:
  UnitConverter/1 -> VHAL_DisChrgPlugErr_enum/1
  DisChrgPlugErr/1 -> UnitConverter/1

== system halin/HAL_IN/CAN3/BMS6/ExtChrgSta ==
  ExtChrgSta : Inport
  UnitConverter : DataTypeConversion  OutDataTypeStr=uint8
  VHAL_ExtChrgSta_enum : Outport
  wires:
  UnitConverter/1 -> VHAL_ExtChrgSta_enum/1
  ExtChrgSta/1 -> UnitConverter/1

== system halin/HAL_IN/CAN3/BMS6/HVBChrgErr ==
  HVBChrgErr : Inport
  UnitConverter : DataTypeConversion  OutDataTypeStr=uint8
  VHAL_HVBChrgErr_enum : Outport
  wires:
  UnitConverter/1 -> VHAL_HVBChrgErr_enum/1
  HVBChrgErr/1 -> UnitConverter/1

== system halin/HAL_IN/CAN3/BMS6/HVBContactorSta ==
  HVBContactorSta : Inport
  UnitConverter : DataTypeConversion  OutDataTypeStr=uint8
  VHAL_HVBContactorSta_flg : Outport
  wires:
  UnitConverter/1 -> VHAL_HVBContactorSta_flg/1
  HVBContactorSta/1 -> UnitConverter/1

== system halin/HAL_IN/CAN3/BMS6/HVBHVILErr ==
  HVBHVILErr : Inport
  UnitConverter : DataTypeConversion  OutDataTypeStr=uint8
  VHAL_HVBHVILErr_flg : Outport
  wires:
  UnitConverter/1 -> VHAL_HVBHVILErr_flg/1
  HVBHVILErr/1 -> UnitConverter/1

== system halin/HAL_IN/CAN3/BMS6/HVBOvrTempErr ==
  HVBOvrTempErr : Inport
  UnitConverter : DataTypeConversion  OutDataTypeStr=uint8
  VHAL_HVBOvrTempErr_flg : Outport
  wires:
  UnitConverter/1 -> VHAL_HVBOvrTempErr_flg/1
  HVBOvrTempErr/1 -> UnitConverter/1

== system halin/HAL_IN/CAN3/BMS6/HVBOvrTempWarn ==
  HVBOvrTempWarn : Inport
  UnitConverter : DataTypeConversion  OutDataTypeStr=uint8
  VHAL_HVBOvrTempWarn_enum : Outport
  wires:
  UnitConverter/1 -> VHAL_HVBOvrTempWarn_enum/1
  HVBOvrTempWarn/1 -> UnitConverter/1

== system halin/HAL_IN/CAN3/BMS6/HVBPreheatPrecoolSta ==
  HVBPreheatPrecoolSta : Inport
  UnitConverter : DataTypeConversion  OutDataTypeStr=uint8
  VHAL_HVBPreheatPrecoolSta_enum : Outport
  wires:
  UnitConverter/1 -> VHAL_HVBPreheatPrecoolSta_enum/1
  HVBPreheatPrecoolSta/1 -> UnitConverter/1

== system halin/HAL_IN/CAN3/BMS6/HVBattReady4Pre ==
  HVBattReady4Pre : Inport
  UnitConverter : DataTypeConversion  OutDataTypeStr=uint8
  VHAL_HVBattReady4Pre_enum : Outport
  wires:
  UnitConverter/1 -> VHAL_HVBattReady4Pre_enum/1
  HVBattReady4Pre/1 -> UnitConverter/1

== system halin/HAL_IN/CAN3/BMS6/HVILSta ==
  HVILSta : Inport
  UnitConverter : DataTypeConversion  OutDataTypeStr=uint8
  VHAL_HVILSta_flg : Outport
  wires:
  UnitConverter/1 -> VHAL_HVILSta_flg/1
  HVILSta/1 -> UnitConverter/1

== system halin/HAL_IN/CAN3/BMS6/V2LSta ==
  V2LSta : Inport
  UnitConverter : DataTypeConversion  OutDataTypeStr=uint8
  VHAL_V2LSta_enum : Outport
  wires:
  UnitConverter/1 -> VHAL_V2LSta_enum/1
  V2LSta/1 -> UnitConverter/1

== system halin/HAL_IN/CAN3/BMS8/MainRlyNegSta ==
  MainRlyNegSta : Inport
  UnitConverter : DataTypeConversion  OutDataTypeStr=uint8
  VHAL_MainRlyNegSta_enum : Outport
  wires:
  UnitConverter/1 -> VHAL_MainRlyNegSta_enum/1
  MainRlyNegSta/1 -> UnitConverter/1

== system halin/HAL_IN/CAN3/BMS8/MainRlyPosSta ==
  MainRlyPosSta : Inport
  UnitConverter : DataTypeConversion  OutDataTypeStr=uint8
  VHAL_MainRlyPosSta_enum : Outport
  wires:
  UnitConverter/1 -> VHAL_MainRlyPosSta_enum/1
  MainRlyPosSta/1 -> UnitConverter/1

== system halin/HAL_IN/CAN3/CCU1/CSCCU1 ==
  CS_CCU1 : Inport
  UnitConverter : DataTypeConversion  OutDataTypeStr=uint8
  VHAL_CSCCU1_enum : Outport
  wires:
  UnitConverter/1 -> VHAL_CSCCU1_enum/1
  CS_CCU1/1 -> UnitConverter/1

== system halin/HAL_IN/CAN3/CCU1/DCDCAuxCur ==
  DCDCAuxCur : Inport
  UnitConverter : DataTypeConversion  OutDataTypeStr=uint16
  convert_in : FVT_lib/hal/convert_in  gain=0.1  offset=0
  VHAL_DCDCAuxCur_A : Outport
  wires:
  convert_in/1 -> VHAL_DCDCAuxCur_A/1
  UnitConverter/1 -> convert_in/1
  DCDCAuxCur/1 -> UnitConverter/1

== system halin/HAL_IN/CAN3/CCU1/DCDCAuxVolt ==
  DCDCAuxVolt : Inport
  UnitConverter : DataTypeConversion  OutDataTypeStr=uint16
  convert_in : FVT_lib/hal/convert_in  gain=0.047  offset=8
  VHAL_DCDCAuxVolt_V : Outport
  wires:
  convert_in/1 -> VHAL_DCDCAuxVolt_V/1
  UnitConverter/1 -> convert_in/1
  DCDCAuxVolt/1 -> UnitConverter/1

== system halin/HAL_IN/CAN3/CCU1/DCDCHVCur ==
  DCDCHVCur : Inport
  UnitConverter : DataTypeConversion  OutDataTypeStr=uint16
  convert_in : FVT_lib/hal/convert_in  gain=0.02  offset=0
  VHAL_DCDCHVCur_A : Outport
  wires:
  convert_in/1 -> VHAL_DCDCHVCur_A/1
  UnitConverter/1 -> convert_in/1
  DCDCHVCur/1 -> UnitConverter/1

== system halin/HAL_IN/CAN3/CCU1/DCDCInVoltInf ==
  DCDCInVoltInf : Inport
  UnitConverter : DataTypeConversion  OutDataTypeStr=uint16
  convert_in : FVT_lib/hal/convert_in  gain=0.25  offset=0
  VHAL_DCDCInVoltInf_V : Outport
  wires:
  convert_in/1 -> VHAL_DCDCInVoltInf_V/1
  UnitConverter/1 -> convert_in/1
  DCDCInVoltInf/1 -> UnitConverter/1

== system halin/HAL_IN/CAN3/CCU1/DCDCPreCompleted ==
  DCDCPreCompleted : Inport
  UnitConverter : DataTypeConversion  OutDataTypeStr=uint8
  VHAL_DCDCPreCompleted_enum : Outport
  wires:
  UnitConverter/1 -> VHAL_DCDCPreCompleted_enum/1
  DCDCPreCompleted/1 -> UnitConverter/1

== system halin/HAL_IN/CAN3/CCU1/OBCDCCurrInf ==
  OBCDCCurrInf : Inport
  UnitConverter : DataTypeConversion  OutDataTypeStr=uint16
  convert_in : FVT_lib/hal/convert_in  gain=0.1  offset=-25.5
  VHAL_OBCDCCurrInf_A : Outport
  wires:
  convert_in/1 -> VHAL_OBCDCCurrInf_A/1
  UnitConverter/1 -> convert_in/1
  OBCDCCurrInf/1 -> UnitConverter/1

== system halin/HAL_IN/CAN3/CCU1/OBCDCVoltInf ==
  OBCDCVoltInf : Inport
  UnitConverter : DataTypeConversion  OutDataTypeStr=uint16
  convert_in : FVT_lib/hal/convert_in  gain=0.3  offset=0
  VHAL_OBCDCVoltInf_V : Outport
  wires:
  convert_in/1 -> VHAL_OBCDCVoltInf_V/1
  UnitConverter/1 -> convert_in/1
  OBCDCVoltInf/1 -> UnitConverter/1

== system halin/HAL_IN/CAN3/CCU1/OBCPreCompleted ==
  OBCPreCompleted : Inport
  UnitConverter : DataTypeConversion  OutDataTypeStr=uint16
  VHAL_OBCPreCompleted_enum : Outport
  wires:
  UnitConverter/1 -> VHAL_OBCPreCompleted_enum/1
  OBCPreCompleted/1 -> UnitConverter/1

== system halin/HAL_IN/CAN3/CCU1/OBCWakeup4Plugin ==
  OBCWakeup4Plugin : Inport
  UnitConverter : DataTypeConversion  OutDataTypeStr=uint8
  VHAL_OBCWakeup4Plugin_flg : Outport
  wires:
  UnitConverter/1 -> VHAL_OBCWakeup4Plugin_flg/1
  OBCWakeup4Plugin/1 -> UnitConverter/1

== system halin/HAL_IN/CAN3/CCU1/RCCCU1 ==
  RC_CCU1 : Inport
  UnitConverter : DataTypeConversion  OutDataTypeStr=uint8
  VHAL_RCCCU1_enum : Outport
  wires:
  UnitConverter/1 -> VHAL_RCCCU1_enum/1
  RC_CCU1/1 -> UnitConverter/1

== system halin/HAL_IN/CAN3/CCU2/CSCCU2 ==
  CS_CCU2 : Inport
  UnitConverter : DataTypeConversion  OutDataTypeStr=uint8
  VHAL_CSCCU2_enum : Outport
  wires:
  UnitConverter/1 -> VHAL_CSCCU2_enum/1
  CS_CCU2/1 -> UnitConverter/1

== system halin/HAL_IN/CAN3/CCU2/DCDCEnaSta ==
  DCDCEnaSta : Inport
  UnitConverter : DataTypeConversion  OutDataTypeStr=uint8
  VHAL_DCDCEnaSta_flg : Outport
  wires:
  UnitConverter/1 -> VHAL_DCDCEnaSta_flg/1
  DCDCEnaSta/1 -> UnitConverter/1

== system halin/HAL_IN/CAN3/CCU2/DCDCFaultSta ==
  DCDCFaultSta : Inport
  UnitConverter : DataTypeConversion  OutDataTypeStr=uint8
  VHAL_DCDCFaultSta_enum : Outport
  wires:
  UnitConverter/1 -> VHAL_DCDCFaultSta_enum/1
  DCDCFaultSta/1 -> UnitConverter/1

== system halin/HAL_IN/CAN3/CCU2/DCDCReady4Pre ==
  DCDCReady4Pre : Inport
  UnitConverter : DataTypeConversion  OutDataTypeStr=uint8
  VHAL_DCDCReady4Pre_flg : Outport
  wires:
  UnitConverter/1 -> VHAL_DCDCReady4Pre_flg/1
  DCDCReady4Pre/1 -> UnitConverter/1

== system halin/HAL_IN/CAN3/CCU2/DCDCTemp ==
  DCDCTemp : Inport
  UnitConverter : DataTypeConversion  OutDataTypeStr=uint8
  convert_in : FVT_lib/hal/convert_in  gain=0.75  offset=-48
  VHAL_DCDCTemp_C : Outport
  wires:
  convert_in/1 -> VHAL_DCDCTemp_C/1
  UnitConverter/1 -> convert_in/1
  DCDCTemp/1 -> UnitConverter/1

== system halin/HAL_IN/CAN3/CCU2/OBCACCurLim ==
  OBC_AC_Cur_Lim : Inport
  UnitConverter : DataTypeConversion  OutDataTypeStr=uint8
  VHAL_OBCACCurLim_enum : Outport
  wires:
  UnitConverter/1 -> VHAL_OBCACCurLim_enum/1
  OBC_AC_Cur_Lim/1 -> UnitConverter/1

== system halin/HAL_IN/CAN3/CCU2/OBCACCurrInf ==
  OBCACCurrInf : Inport
  UnitConverter : DataTypeConversion  OutDataTypeStr=uint16
  convert_in : FVT_lib/hal/convert_in  gain=0.125  offset=-40
  VHAL_OBCACCurrInf_A : Outport
  wires:
  convert_in/1 -> VHAL_OBCACCurrInf_A/1
  UnitConverter/1 -> convert_in/1
  OBCACCurrInf/1 -> UnitConverter/1

== system halin/HAL_IN/CAN3/CCU2/OBCACVoltInf ==
  OBCACVoltInf : Inport
  UnitConverter : DataTypeConversion  OutDataTypeStr=uint16
  convert_in : FVT_lib/hal/convert_in  gain=0.1  offset=0
  VHAL_OBCACVoltInf_V : Outport
  wires:
  convert_in/1 -> VHAL_OBCACVoltInf_V/1
  UnitConverter/1 -> convert_in/1
  OBCACVoltInf/1 -> UnitConverter/1

== system halin/HAL_IN/CAN3/CCU2/OBCEnaSta ==
  OBCEnaSta : Inport
  UnitConverter : DataTypeConversion  OutDataTypeStr=uint8
  VHAL_OBCEnaSta_flg : Outport
  wires:
  UnitConverter/1 -> VHAL_OBCEnaSta_flg/1
  OBCEnaSta/1 -> UnitConverter/1

== system halin/HAL_IN/CAN3/CCU2/OBCFaultSta ==
  OBCFaultSta : Inport
  UnitConverter : DataTypeConversion  OutDataTypeStr=uint8
  VHAL_OBCFaultSta_enum : Outport
  wires:
  UnitConverter/1 -> VHAL_OBCFaultSta_enum/1
  OBCFaultSta/1 -> UnitConverter/1

== system halin/HAL_IN/CAN3/CCU2/OBCPluginSta ==
  OBCPluginSta : Inport
  UnitConverter : DataTypeConversion  OutDataTypeStr=uint8
  VHAL_OBCPluginSta_flg : Outport
  wires:
  UnitConverter/1 -> VHAL_OBCPluginSta_flg/1
  OBCPluginSta/1 -> UnitConverter/1

== system halin/HAL_IN/CAN3/CCU2/OBCReady4Pre ==
  OBCReady4Pre : Inport
  UnitConverter : DataTypeConversion  OutDataTypeStr=uint8
  VHAL_OBCReady4Pre_flg : Outport
  wires:
  UnitConverter/1 -> VHAL_OBCReady4Pre_flg/1
  OBCReady4Pre/1 -> UnitConverter/1

== system halin/HAL_IN/CAN3/CCU2/OBCTemp ==
  OBCTemp : Inport
  UnitConverter : DataTypeConversion  OutDataTypeStr=uint16
  convert_in : FVT_lib/hal/convert_in  gain=0.3  offset=-48
  VHAL_OBCTemp_C : Outport
  wires:
  convert_in/1 -> VHAL_OBCTemp_C/1
  UnitConverter/1 -> convert_in/1
  OBCTemp/1 -> UnitConverter/1

== system halin/HAL_IN/CAN3/CCU2/OBCV2LSta ==
  OBCV2LSta : Inport
  UnitConverter : DataTypeConversion  OutDataTypeStr=uint8
  VHAL_OBCV2LSta_enum : Outport
  wires:
  UnitConverter/1 -> VHAL_OBCV2LSta_enum/1
  OBCV2LSta/1 -> UnitConverter/1

== system halin/HAL_IN/CAN3/CCU2/RCCCU2 ==
  RC_CCU2 : Inport
  UnitConverter : DataTypeConversion  OutDataTypeStr=uint8
  VHAL_RCCCU2_enum : Outport
  wires:
  UnitConverter/1 -> VHAL_RCCCU2_enum/1
  RC_CCU2/1 -> UnitConverter/1

== system halin/HAL_IN/CAN3/EBM1/EBMErrSta ==
  EBMErrSta : Inport
  UnitConverter : DataTypeConversion  OutDataTypeStr=uint8
  VHAL_EBMErrSta_enum : Outport
  wires:
  UnitConverter/1 -> VHAL_EBMErrSta_enum/1
  EBMErrSta/1 -> UnitConverter/1

== system halin/HAL_IN/CAN3/EBM1/EBMRLampSta ==
  EBMRLampSta : Inport
  UnitConverter : DataTypeConversion  OutDataTypeStr=uint8
  VHAL_EBMRLampSta_enum : Outport
  wires:
  UnitConverter/1 -> VHAL_EBMRLampSta_enum/1
  EBMRLampSta/1 -> UnitConverter/1

== system halin/HAL_IN/CAN3/MCU_B_F1/FrActvDmpDisabSta ==
  Fr_ActvDmpDisabSta : Inport
  UnitConverter : DataTypeConversion  OutDataTypeStr=uint8
  VHAL_FrActvDmpDisabSta_flg : Outport
  wires:
  UnitConverter/1 -> VHAL_FrActvDmpDisabSta_flg/1
  Fr_ActvDmpDisabSta/1 -> UnitConverter/1

== system halin/HAL_IN/CAN3/MCU_B_F1/FrEDUDrtSta ==
  Fr_EDUDrtSta : Inport
  UnitConverter : DataTypeConversion  OutDataTypeStr=uint8
  VHAL_FrEDUDrtSta_flg : Outport
  wires:
  UnitConverter/1 -> VHAL_FrEDUDrtSta_flg/1
  Fr_EDUDrtSta/1 -> UnitConverter/1

== system halin/HAL_IN/CAN3/MCU_B_F1/FrEDUOpratingSta ==
  Fr_EDUOpratingSta : Inport
  UnitConverter : DataTypeConversion  OutDataTypeStr=uint8
  VHAL_FrEDUOpratingSta_flg : Outport
  wires:
  UnitConverter/1 -> VHAL_FrEDUOpratingSta_flg/1
  Fr_EDUOpratingSta/1 -> UnitConverter/1

== system halin/HAL_IN/CAN3/MCU_B_F1/FrEDURealTMTq ==
  Fr_EDURealTMTq : Inport
  UnitConverter : DataTypeConversion  OutDataTypeStr=uint16
  convert_in : FVT_lib/hal/convert_in  gain=1  offset=-1022
  VHAL_FrEDURealTMTq_Nm : Outport
  wires:
  convert_in/1 -> VHAL_FrEDURealTMTq_Nm/1
  UnitConverter/1 -> convert_in/1
  Fr_EDURealTMTq/1 -> UnitConverter/1

== system halin/HAL_IN/CAN3/MCU_B_F1/FrEDURotateDirction ==
  Fr_EDURotateDirction : Inport
  UnitConverter : DataTypeConversion  OutDataTypeStr=uint8
  VHAL_FrEDURotateDirction_enum : Outport
  wires:
  UnitConverter/1 -> VHAL_FrEDURotateDirction_enum/1
  Fr_EDURotateDirction/1 -> UnitConverter/1

== system halin/HAL_IN/CAN3/MCU_B_F1/FrEDUTqReqFbk ==
  Fr_EDUTqReqFbk : Inport
  UnitConverter : DataTypeConversion  OutDataTypeStr=uint16
  convert_in : FVT_lib/hal/convert_in  gain=1  offset=-1022
  VHAL_FrEDUTqReqFbk_Nm : Outport
  wires:
  convert_in/1 -> VHAL_FrEDUTqReqFbk_Nm/1
  UnitConverter/1 -> convert_in/1
  Fr_EDUTqReqFbk/1 -> UnitConverter/1

== system halin/HAL_IN/CAN3/MCU_B_F1/FrMCUBAT ==
  Fr_MCUBAT : Inport
  UnitConverter : DataTypeConversion  OutDataTypeStr=uint8
  convert_in : FVT_lib/hal/convert_in  gain=0.1  offset=0
  VHAL_FrMCUBAT_V : Outport
  wires:
  convert_in/1 -> VHAL_FrMCUBAT_V/1
  UnitConverter/1 -> convert_in/1
  Fr_MCUBAT/1 -> UnitConverter/1

== system halin/HAL_IN/CAN3/MCU_B_F1/FrMCUDCBusCurr ==
  Fr_MCUDCBusCurr : Inport
  UnitConverter : DataTypeConversion  OutDataTypeStr=uint16
  convert_in : FVT_lib/hal/convert_in  gain=0.1  offset=-1500
  VHAL_FrMCUDCBusCurr_A : Outport
  wires:
  convert_in/1 -> VHAL_FrMCUDCBusCurr_A/1
  UnitConverter/1 -> convert_in/1
  Fr_MCUDCBusCurr/1 -> UnitConverter/1

== system halin/HAL_IN/CAN3/MCU_B_F1/FrMCUDCBusVolt ==
  Fr_MCUDCBusVolt : Inport
  UnitConverter : DataTypeConversion  OutDataTypeStr=uint16
  convert_in : FVT_lib/hal/convert_in  gain=0.1  offset=0
  VHAL_FrMCUDCBusVolt_V : Outport
  wires:
  convert_in/1 -> VHAL_FrMCUDCBusVolt_V/1
  UnitConverter/1 -> convert_in/1
  Fr_MCUDCBusVolt/1 -> UnitConverter/1

== system halin/HAL_IN/CAN3/MCU_B_F1/FrMCUDischrgSta ==
  Fr_MCUDischrgSta : Inport
  UnitConverter : DataTypeConversion  OutDataTypeStr=uint8
  VHAL_FrMCUDischrgSta_flg : Outport
  wires:
  UnitConverter/1 -> VHAL_FrMCUDischrgSta_flg/1
  Fr_MCUDischrgSta/1 -> UnitConverter/1

== system halin/HAL_IN/CAN3/MCU_B_F1/FrMCUEnaSta ==
  Fr_MCUEnaSta : Inport
  UnitConverter : DataTypeConversion  OutDataTypeStr=uint8
  VHAL_FrMCUEnaSta_flg : Outport
  wires:
  UnitConverter/1 -> VHAL_FrMCUEnaSta_flg/1
  Fr_MCUEnaSta/1 -> UnitConverter/1

== system halin/HAL_IN/CAN3/MCU_B_F1/FrMCUErr ==
  Fr_MCUErr : Inport
  UnitConverter : DataTypeConversion  OutDataTypeStr=uint8
  VHAL_FrMCUErr_enum : Outport
  wires:
  UnitConverter/1 -> VHAL_FrMCUErr_enum/1
  Fr_MCUErr/1 -> UnitConverter/1

== system halin/HAL_IN/CAN3/MCU_B_F1/FrMCUIGNsta ==
  Fr_MCUIGN_sta : Inport
  UnitConverter : DataTypeConversion  OutDataTypeStr=uint8
  VHAL_FrMCUIGNsta_flg : Outport
  wires:
  UnitConverter/1 -> VHAL_FrMCUIGNsta_flg/1
  Fr_MCUIGN_sta/1 -> UnitConverter/1

== system halin/HAL_IN/CAN3/MCU_B_F1/FrMCUReady ==
  Fr_MCUReady : Inport
  UnitConverter : DataTypeConversion  OutDataTypeStr=uint8
  VHAL_FrMCUReady_flg : Outport
  wires:
  UnitConverter/1 -> VHAL_FrMCUReady_flg/1
  Fr_MCUReady/1 -> UnitConverter/1

== system halin/HAL_IN/CAN3/MCU_B_F1/FrMCUReady4Pre ==
  Fr_MCUReady4Pre : Inport
  UnitConverter : DataTypeConversion  OutDataTypeStr=uint8
  VHAL_FrMCUReady4Pre_flg : Outport
  wires:
  UnitConverter/1 -> VHAL_FrMCUReady4Pre_flg/1
  Fr_MCUReady4Pre/1 -> UnitConverter/1

== system halin/HAL_IN/CAN3/MCU_B_F1/FrMCUSysSta ==
  Fr_MCUSysSta : Inport
  UnitConverter : DataTypeConversion  OutDataTypeStr=uint8
  VHAL_FrMCUSysSta_enum : Outport
  wires:
  UnitConverter/1 -> VHAL_FrMCUSysSta_enum/1
  Fr_MCUSysSta/1 -> UnitConverter/1

== system halin/HAL_IN/CAN3/MCU_B_F1/FrMCUTemp ==
  Fr_MCUTemp : Inport
  UnitConverter : DataTypeConversion  OutDataTypeStr=uint16
  convert_in : FVT_lib/hal/convert_in  gain=1  offset=-40
  VHAL_FrMCUTemp_C : Outport
  wires:
  convert_in/1 -> VHAL_FrMCUTemp_C/1
  UnitConverter/1 -> convert_in/1
  Fr_MCUTemp/1 -> UnitConverter/1

== system halin/HAL_IN/CAN3/MCU_B_F1/FrMotorAvailTq ==
  Fr_MotorAvailTq : Inport
  UnitConverter : DataTypeConversion  OutDataTypeStr=uint16
  VHAL_FrMotorAvailTq_Nm : Outport
  wires:
  UnitConverter/1 -> VHAL_FrMotorAvailTq_Nm/1
  Fr_MotorAvailTq/1 -> UnitConverter/1

== system halin/HAL_IN/CAN3/MCU_B_F1/FrRegenAvailTq ==
  Fr_RegenAvailTq : Inport
  UnitConverter : DataTypeConversion  OutDataTypeStr=uint16
  convert_in : FVT_lib/hal/convert_in  gain=1  offset=-1022
  VHAL_FrRegenAvailTq_Nm : Outport
  wires:
  convert_in/1 -> VHAL_FrRegenAvailTq_Nm/1
  UnitConverter/1 -> convert_in/1
  Fr_RegenAvailTq/1 -> UnitConverter/1

== system halin/HAL_IN/CAN3/MCU_B_F1/FrTMSpd ==
  Fr_TMSpd : Inport
  UnitConverter : DataTypeConversion  OutDataTypeStr=uint16
  convert_in : FVT_lib/hal/convert_in  gain=1  offset=-18000
  VHAL_FrTMSpd_rpm : Outport
  wires:
  convert_in/1 -> VHAL_FrTMSpd_rpm/1
  UnitConverter/1 -> convert_in/1
  Fr_TMSpd/1 -> UnitConverter/1

== system halin/HAL_IN/CAN3/MCU_B_F1/FrTMTemp ==
  Fr_TMTemp : Inport
  UnitConverter : DataTypeConversion  OutDataTypeStr=uint16
  convert_in : FVT_lib/hal/convert_in  gain=1  offset=-40
  VHAL_FrTMTemp_C : Outport
  wires:
  convert_in/1 -> VHAL_FrTMTemp_C/1
  UnitConverter/1 -> convert_in/1
  Fr_TMTemp/1 -> UnitConverter/1

== system halin/HAL_IN/CAN3/MCU_B_F1/FrTMid ==
  Fr_TMid : Inport
  UnitConverter : DataTypeConversion  OutDataTypeStr=uint16
  convert_in : FVT_lib/hal/convert_in  gain=0.1  offset=-1500
  VHAL_FrTMid_A : Outport
  wires:
  convert_in/1 -> VHAL_FrTMid_A/1
  UnitConverter/1 -> convert_in/1
  Fr_TMid/1 -> UnitConverter/1

== system halin/HAL_IN/CAN3/MCU_B_F1/FrTMiq ==
  Fr_TMiq : Inport
  UnitConverter : DataTypeConversion  OutDataTypeStr=uint16
  convert_in : FVT_lib/hal/convert_in  gain=0.1  offset=-1500
  VHAL_FrTMiq_A : Outport
  wires:
  convert_in/1 -> VHAL_FrTMiq_A/1
  UnitConverter/1 -> convert_in/1
  Fr_TMiq/1 -> UnitConverter/1

== system halin/HAL_IN/CAN3/MCU_B_F1/MCUWarnF ==
  MCUWarn_F : Inport
  UnitConverter : DataTypeConversion  OutDataTypeStr=uint8
  VHAL_MCUWarnF_enum : Outport
  wires:
  UnitConverter/1 -> VHAL_MCUWarnF_enum/1
  MCUWarn_F/1 -> UnitConverter/1

== system halin/HAL_IN/CAN3/MCU_B_F2/FrCoolanttempReq ==
  Fr_CoolanttempReq : Inport
  UnitConverter : DataTypeConversion  OutDataTypeStr=uint16
  convert_in : FVT_lib/hal/convert_in  gain=1  offset=-40
  VHAL_FrCoolanttempReq_C : Outport
  wires:
  convert_in/1 -> VHAL_FrCoolanttempReq_C/1
  UnitConverter/1 -> convert_in/1
  Fr_CoolanttempReq/1 -> UnitConverter/1

== system halin/HAL_IN/CAN3/MCU_B_F2/FrFailcode1 ==
  Fr_Failcode1 : Inport
  UnitConverter : DataTypeConversion  OutDataTypeStr=uint8
  VHAL_FrFailcode1_enum : Outport
  wires:
  UnitConverter/1 -> VHAL_FrFailcode1_enum/1
  Fr_Failcode1/1 -> UnitConverter/1

== system halin/HAL_IN/CAN3/MCU_B_F2/FrFailcode2 ==
  Fr_Failcode2 : Inport
  UnitConverter : DataTypeConversion  OutDataTypeStr=uint8
  VHAL_FrFailcode2_enum : Outport
  wires:
  UnitConverter/1 -> VHAL_FrFailcode2_enum/1
  Fr_Failcode2/1 -> UnitConverter/1

== system halin/HAL_IN/CAN3/MCU_B_F2/FrFailcodehistory1 ==
  Fr_Failcodehistory1 : Inport
  UnitConverter : DataTypeConversion  OutDataTypeStr=uint8
  VHAL_FrFailcodehistory1_enum : Outport
  wires:
  UnitConverter/1 -> VHAL_FrFailcodehistory1_enum/1
  Fr_Failcodehistory1/1 -> UnitConverter/1

== system halin/HAL_IN/CAN3/MCU_B_F2/FrFailcodehistory2 ==
  Fr_Failcodehistory2 : Inport
  UnitConverter : DataTypeConversion  OutDataTypeStr=uint8
  VHAL_FrFailcodehistory2_enum : Outport
  wires:
  UnitConverter/1 -> VHAL_FrFailcodehistory2_enum/1
  Fr_Failcodehistory2/1 -> UnitConverter/1

== system halin/HAL_IN/CAN3/MCU_B_F2/FrLLCTemp ==
  Fr_LLCTemp : Inport
  UnitConverter : DataTypeConversion  OutDataTypeStr=uint16
  convert_in : FVT_lib/hal/convert_in  gain=1  offset=-40
  VHAL_FrLLCTemp_C : Outport
  wires:
  convert_in/1 -> VHAL_FrLLCTemp_C/1
  UnitConverter/1 -> convert_in/1
  Fr_LLCTemp/1 -> UnitConverter/1

== system halin/HAL_IN/CAN3/MCU_B_F2/FrLLCflowReq ==
  Fr_LLCflowReq : Inport
  UnitConverter : DataTypeConversion  OutDataTypeStr=uint8
  convert_in : FVT_lib/hal/convert_in  gain=0.25  offset=0
  VHAL_FrLLCflowReq_Lpmin : Outport
  wires:
  convert_in/1 -> VHAL_FrLLCflowReq_Lpmin/1
  UnitConverter/1 -> convert_in/1
  Fr_LLCflowReq/1 -> UnitConverter/1

== system halin/HAL_IN/CAN3/MCU_B_F2/FrMCUHWVer ==
  Fr_MCU_HW_Ver : Inport
  UnitConverter : DataTypeConversion  OutDataTypeStr=uint16
  VHAL_FrMCUHWVer_enum : Outport
  wires:
  UnitConverter/1 -> VHAL_FrMCUHWVer_enum/1
  Fr_MCU_HW_Ver/1 -> UnitConverter/1

== system halin/HAL_IN/CAN3/MCU_B_F2/FrMCUSWVer ==
  Fr_MCU_SW_Ver : Inport
  UnitConverter : DataTypeConversion  OutDataTypeStr=uint16
  VHAL_FrMCUSWVer_enum : Outport
  wires:
  UnitConverter/1 -> VHAL_FrMCUSWVer_enum/1
  Fr_MCU_SW_Ver/1 -> UnitConverter/1

== system halin/HAL_IN/CAN3/MCU_B_F2/FrMCUTempWarn ==
  Fr_MCUTempWarn : Inport
  UnitConverter : DataTypeConversion  OutDataTypeStr=uint8
  VHAL_FrMCUTempWarn_enum : Outport
  wires:
  UnitConverter/1 -> VHAL_FrMCUTempWarn_enum/1
  Fr_MCUTempWarn/1 -> UnitConverter/1

== system halin/HAL_IN/CAN3/MCU_B_F2/FrTMTempWarn ==
  Fr_TMTempWarn : Inport
  UnitConverter : DataTypeConversion  OutDataTypeStr=uint8
  VHAL_FrTMTempWarn_enum : Outport
  wires:
  UnitConverter/1 -> VHAL_FrTMTempWarn_enum/1
  Fr_TMTempWarn/1 -> UnitConverter/1

== system halin/HAL_IN/CAN3/MCU_B_F2/MCUBFLLCTempWarnSta ==
  MCU_B_F_LLCTempWarn_Sta : Inport
  UnitConverter : DataTypeConversion  OutDataTypeStr=uint8
  VHAL_MCUBFLLCTempWarnSta_enum : Outport
  wires:
  UnitConverter/1 -> VHAL_MCUBFLLCTempWarnSta_enum/1
  MCU_B_F_LLCTempWarn_Sta/1 -> UnitConverter/1

== system halin/HAL_IN/CAN3/MCU_B_R1/MCUWarnR ==
  MCUWarn_R : Inport
  UnitConverter : DataTypeConversion  OutDataTypeStr=uint8
  VHAL_MCUWarnR_enum : Outport
  wires:
  UnitConverter/1 -> VHAL_MCUWarnR_enum/1
  MCUWarn_R/1 -> UnitConverter/1

== system halin/HAL_IN/CAN3/MCU_B_R1/RrActvDmpDisabSta ==
  Rr_ActvDmpDisabSta : Inport
  UnitConverter : DataTypeConversion  OutDataTypeStr=uint8
  VHAL_RrActvDmpDisabSta_flg : Outport
  wires:
  UnitConverter/1 -> VHAL_RrActvDmpDisabSta_flg/1
  Rr_ActvDmpDisabSta/1 -> UnitConverter/1

== system halin/HAL_IN/CAN3/MCU_B_R1/RrEDUDrtSta ==
  Rr_EDUDrtSta : Inport
  UnitConverter : DataTypeConversion  OutDataTypeStr=uint8
  VHAL_RrEDUDrtSta_flg : Outport
  wires:
  UnitConverter/1 -> VHAL_RrEDUDrtSta_flg/1
  Rr_EDUDrtSta/1 -> UnitConverter/1

== system halin/HAL_IN/CAN3/MCU_B_R1/RrEDUOpratingSta ==
  Rr_EDUOpratingSta : Inport
  UnitConverter : DataTypeConversion  OutDataTypeStr=uint8
  VHAL_RrEDUOpratingSta_flg : Outport
  wires:
  UnitConverter/1 -> VHAL_RrEDUOpratingSta_flg/1
  Rr_EDUOpratingSta/1 -> UnitConverter/1

== system halin/HAL_IN/CAN3/MCU_B_R1/RrEDURealTMTq ==
  Rr_EDURealTMTq : Inport
  UnitConverter : DataTypeConversion  OutDataTypeStr=uint16
  convert_in : FVT_lib/hal/convert_in  gain=1  offset=-1022
  VHAL_RrEDURealTMTq_Nm : Outport
  wires:
  convert_in/1 -> VHAL_RrEDURealTMTq_Nm/1
  UnitConverter/1 -> convert_in/1
  Rr_EDURealTMTq/1 -> UnitConverter/1

== system halin/HAL_IN/CAN3/MCU_B_R1/RrEDURotateDirction ==
  Rr_EDURotateDirction : Inport
  UnitConverter : DataTypeConversion  OutDataTypeStr=uint8
  VHAL_RrEDURotateDirction_enum : Outport
  wires:
  UnitConverter/1 -> VHAL_RrEDURotateDirction_enum/1
  Rr_EDURotateDirction/1 -> UnitConverter/1

== system halin/HAL_IN/CAN3/MCU_B_R1/RrEDUTqReqFbk ==
  Rr_EDUTqReqFbk : Inport
  UnitConverter : DataTypeConversion  OutDataTypeStr=uint16
  convert_in : FVT_lib/hal/convert_in  gain=1  offset=-1022
  VHAL_RrEDUTqReqFbk_Nm : Outport
  wires:
  convert_in/1 -> VHAL_RrEDUTqReqFbk_Nm/1
  UnitConverter/1 -> convert_in/1
  Rr_EDUTqReqFbk/1 -> UnitConverter/1

== system halin/HAL_IN/CAN3/MCU_B_R1/RrMCUBAT ==
  Rr_MCUBAT : Inport
  UnitConverter : DataTypeConversion  OutDataTypeStr=uint8
  convert_in : FVT_lib/hal/convert_in  gain=0.1  offset=0
  VHAL_RrMCUBAT_V : Outport
  wires:
  convert_in/1 -> VHAL_RrMCUBAT_V/1
  UnitConverter/1 -> convert_in/1
  Rr_MCUBAT/1 -> UnitConverter/1
